simulink model "Lab_4"  (Simulink 9.1)
settings: Solver=VariableStepAuto  StartTime=0.0  StopTime=simulation_time  MaxStep=0.1
values from neighbouring files (symbols this model uses):
  a = (r_a + r_p)/2    (= 7178)    [main.m]
  i = 0    [main.m]
  I_1 = 0.0109    [main.m]
  I_2 = 0.0504    [main.m]
  I_3 = 0.055    [main.m]
  mu = 398600    [main.m]
  OMG = 0    [main.m]
  omg = 0    [main.m]
  phi_0 = 0    [main.m]
  psi_0 = 0    [main.m]
  q_c = [0; 1; 0; 0]    [main.m]
  theta = 0    [main.m]
  theta_0 = 0    [main.m]
  w1_0 = 0.02    [main.m]
  w2_0 = 0.01    [main.m]
  w3_0 = 0.05    [main.m]
undefined symbols (not defined in the file or in its folder): DCM_0, q_0
libraries: dspmathops x2, sharedutil x1
settings Model: SuppressorTable=22 serialization::archive 11 0 6 0 0 0 1 0  Creator=fcuzzocrea  LastModifiedBy=fcuzzocrea
settings DataIOCC: SaveFormat=Dataset
settings OptimizationCC: LifeSpan=auto
settings DebuggingCC: UnderspecifiedInitializationDetection=Simplified  MergeDetectMultiDrivingBlocksExec=error  SFUnexpectedBacktrackingDiag=error  SFNoUnconditionalDefaultTransitionDiag=error  SFExecutionAtInitializationDiag=warning
settings HardwareCC: ProdBitPerPointer=64  ProdBitPerSizeT=64  ProdBitPerPtrDiffT=64  ProdLargestAtomicFloat=Float  ProdIntDivRoundTo=Zero  ProdEndianess=LittleEndian  ProdWordSize=64  ProdHWDeviceType=Intel->x86-64 (Windows64)
settings ModelReferenceCC: PropagateSignalLabelsOutOfModel=on
settings CodeAppCC: StateflowObjectComments=off
settings GRTTargetCC: TargetLangStandard=C99 (ISO)  CombineOutputUpdateFcns=on  GRTInterface=off
settings ConfigComp: CovMetricSettings=dwe  CovHtmlReporting=off  CovSaveCumulativeToWorkspaceVar=off  CovSaveSingleToWorkspaceVar=off  CovExternalEMLEnable=on

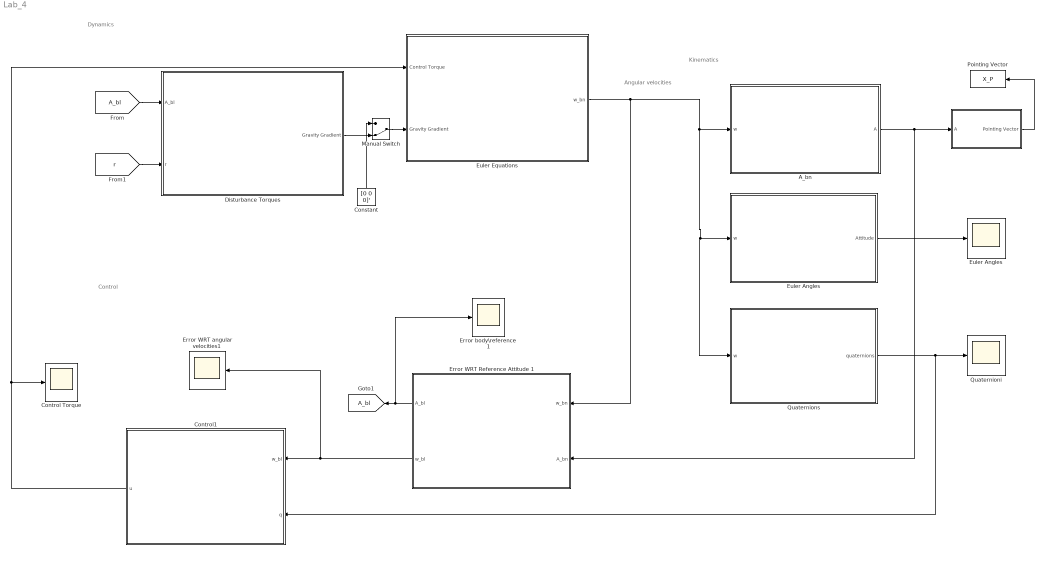
== system Lab_4 ==
  note: Dynamics
  note: Kinematics
  note: Angular velocities
  note: Control
  " " : Subsystem
  A_bn : Subsystem
  Constant : Constant  Value=[0 0 0]'
  "Control Torque " : Scope
  Control1 : Subsystem
  Disturbance Torques : Subsystem
  Error WRT Reference Attitude 1 : Subsystem
  Error WRT angular velocities1 : Scope
  Error body\reference  1 : Scope
  "Euler Angles " : Subsystem
  "Euler Angles  " : Scope
  "Euler Equations " : Subsystem
  Manual Switch : ManualSwitch  CurrentSetting=0
  "Pointing Vector " : ToWorkspace  VariableName=X_P  SampleTime=-1
  "Quaternioni " : Scope
  Quaternions : Subsystem
  tag scope: A_bl=global
  wires:
  " "/1("Pointing Vector ") -> "Pointing Vector "/1
  "Euler Angles "/1(Attitude) -> "Euler Angles  "/1
  [A_bl] -> Disturbance Torques/1(A_bl)
  [r] -> Disturbance Torques/2(r)
  Manual Switch/1 -> "Euler Equations "/2(Gravity Gradient)
  Constant/1 -> Manual Switch/1
  Disturbance Torques/1("Gravity Gradient ") -> Manual Switch/2
  Error WRT Reference Attitude 1/2(w_bl) -> Error WRT angular velocities1/1, Control1/1(w_bl)
  Quaternions/1(quaternions) -> Control1/2(q), "Quaternioni "/1
  A_bn/1(A) -> Error WRT Reference Attitude 1/2(A_bn), " "/1(A)
  Error WRT Reference Attitude 1/1(A_bl) -> Error body\reference  1/1, [A_bl]
  "Euler Equations "/1(w_bn) -> Error WRT Reference Attitude 1/1(w_bn), A_bn/1(w), Quaternions/1(w), "Euler Angles "/1(w)
  Control1/1(u) -> "Euler Equations "/1(Control Torque), "Control Torque "/1

== system Lab_4/  ==
  A : Inport
  Constant3 : Constant  Value=[1 0 0]'  VectorParams1D=off
  Math Function : Math  Operator=transpose  SaturateOnIntegerOverflow=on
  Product1 : Product  Multiplication=Matrix(*)
  "Pointing Vector " : Outport
  wires:
  Constant3/1 -> Product1/2
  Math Function/1 -> Product1/1
  A/1 -> Math Function/1
  Product1/1 -> "Pointing Vector "/1

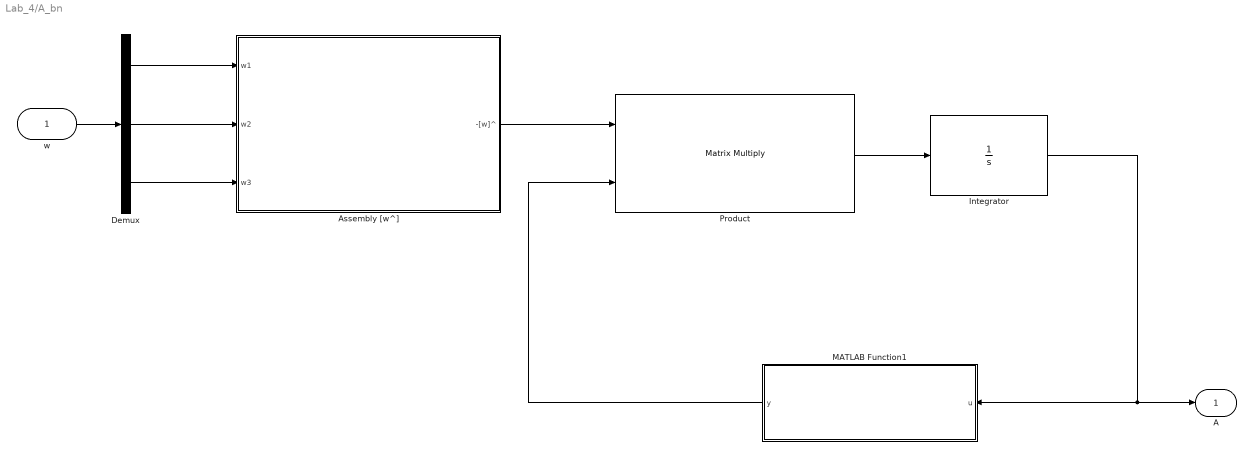
== system Lab_4/A_bn ==
  w : Inport  Unit=rad/s  PortDimensions=3
  "Assembly [w^] " : Subsystem
  Demux : Demux  Outputs=3
  Integrator : Integrator  InitialCondition=DCM_0
  MATLAB Function1 : MATLAB Function  TreatAsAtomicUnit=on
  Product : Product  Multiplication=Matrix(*)
  A : Outport
  wires:
  Product/1 -> Integrator/1
  Integrator/1 -> A/1, MATLAB Function1/1(u)
  w/1 -> Demux/1
  Demux/1 -> "Assembly [w^] "/1(w1)
  Demux/2 -> "Assembly [w^] "/2(w2)
  Demux/3 -> "Assembly [w^] "/3(w3)
  "Assembly [w^] "/1(-[w]^) -> Product/1
  MATLAB Function1/1(y) -> Product/2

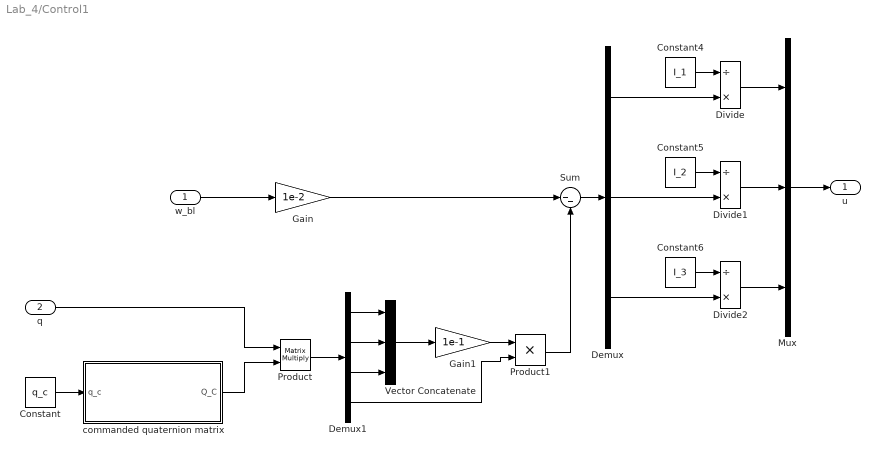
== system Lab_4/Control1 ==
  w_bl : Inport
  q : Inport  Port=2
  Constant : Constant  Value=q_c
  Constant4 : Constant  Value=I_1
  Constant5 : Constant  Value=I_2
  Constant6 : Constant  Value=I_3
  Demux : Demux  Outputs=3
  Demux1 : Demux
  Divide : Product  Inputs=/*
  Divide1 : Product  Inputs=/*
  Divide2 : Product  Inputs=/*
  Gain : Gain  Gain=1e-2
  Gain1 : Gain  Gain=1e-1
  Mux : Mux  Inputs=3
  Product : Product  Multiplication=Matrix(*)
  Product1 : Product
  Sum : Sum  Inputs=|--
  Vector Concatenate : Concatenate  NumInputs=3
  commanded quaternion matrix : MATLAB Function  TreatAsAtomicUnit=on
  u : Outport
  wires:
  w_bl/1 -> Gain/1
  Divide/1 -> Mux/1
  Constant4/1 -> Divide/1
  Constant5/1 -> Divide1/1
  Divide1/1 -> Mux/2
  Constant6/1 -> Divide2/1
  Divide2/1 -> Mux/3
  Demux/2 -> Divide1/2
  Demux/1 -> Divide/2
  Mux/1 -> u/1
  Demux/3 -> Divide2/2
  Constant/1 -> commanded quaternion matrix/1(q_c)
  q/1 -> Product/1
  commanded quaternion matrix/1(Q_C) -> Product/2
  Gain/1 -> Sum/1
  Sum/1 -> Demux/1
  Product/1 -> Demux1/1
  Demux1/4 -> Product1/2
  Demux1/1 -> Vector Concatenate/1
  Demux1/2 -> Vector Concatenate/2
  Demux1/3 -> Vector Concatenate/3
  Vector Concatenate/1 -> Gain1/1
  Gain1/1 -> Product1/1
  Product1/1 -> Sum/2

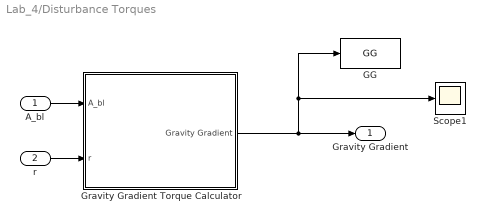
== system Lab_4/Disturbance Torques ==
  A_bl : Inport
  r : Inport  Port=2
  GG : ToWorkspace  VariableName=GG  SampleTime=-1
  Gravity Gradient Torque Calculator : Subsystem
  Scope1 : Scope
  "Gravity Gradient " : Outport
  wires:
  A_bl/1 -> Gravity Gradient Torque Calculator/1(A_bl)
  r/1 -> Gravity Gradient Torque Calculator/2(r)
  Gravity Gradient Torque Calculator/1(Gravity Gradient) -> Scope1/1, GG/1, "Gravity Gradient "/1

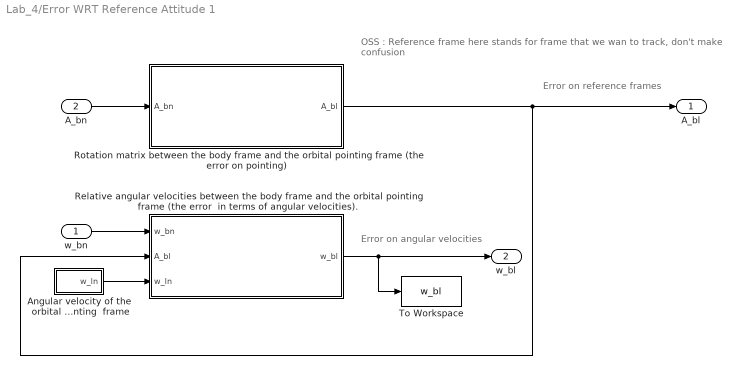
== system Lab_4/Error WRT Reference Attitude 1 ==
  note: Error on angular velocities
  note: Error on reference frames
  note: OSS : Reference frame here stands for frame that we wan to track, don't make confusion
  w_bn : Inport
  A_bn : Inport  Port=2
  Angular velocity of the  orbital pointing  frame : Subsystem
  Relative angular velocities between the body frame and the orbital pointing frame (the error  in terms of angular velocities). : Subsystem
  Rotation matrix between the body frame and the orbital pointing frame (the error on pointing) : Subsystem
  To Workspace : ToWorkspace  VariableName=w_bl  SampleTime=-1
  A_bl : Outport
  w_bl : Outport  Port=2
  wires:
  A_bn/1 -> Rotation matrix between the body frame and the orbital pointing frame (the error on pointing)/1("A_bn ")
  w_bn/1 -> Relative angular velocities between the body frame and the orbital pointing frame (the error  in terms of angular velocities)./1(w_bn)
  Rotation matrix between the body frame and the orbital pointing frame (the error on pointing)/1("A_bl   ") -> A_bl/1, Relative angular velocities between the body frame and the orbital pointing frame (the error  in terms of angular velocities)./2("A_bl ")
  Angular velocity of the  orbital pointing  frame/1(w_ln) -> Relative angular velocities between the body frame and the orbital pointing frame (the error  in terms of angular velocities)./3("w_ln ")
  Relative angular velocities between the body frame and the orbital pointing frame (the error  in terms of angular velocities)./1(w_bl) -> To Workspace/1, w_bl/1

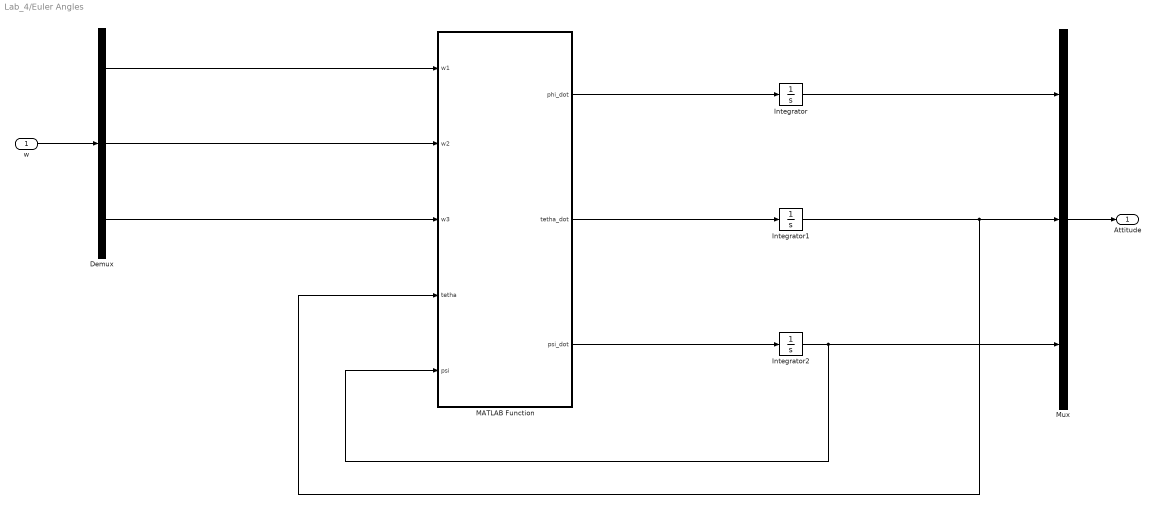
== system Lab_4/Euler Angles  ==
  w : Inport
  Demux : Demux  Outputs=3
  Integrator : Integrator  InitialCondition=phi_0
  Integrator1 : Integrator  InitialCondition=theta_0
  Integrator2 : Integrator  InitialCondition=psi_0
  MATLAB Function : MATLAB Function  TreatAsAtomicUnit=on
  Mux : Mux  Inputs=3
  Attitude : Outport
  wires:
  Demux/1 -> MATLAB Function/1(w1)
  Demux/2 -> MATLAB Function/2(w2)
  Demux/3 -> MATLAB Function/3(w3)
  MATLAB Function/1(phi_dot) -> Integrator/1
  MATLAB Function/2(tetha_dot) -> Integrator1/1
  MATLAB Function/3(psi_dot) -> Integrator2/1
  Integrator/1 -> Mux/1
  Integrator1/1 -> Mux/2, MATLAB Function/4(tetha)
  Mux/1 -> Attitude/1
  Integrator2/1 -> MATLAB Function/5(psi), Mux/3
  w/1 -> Demux/1

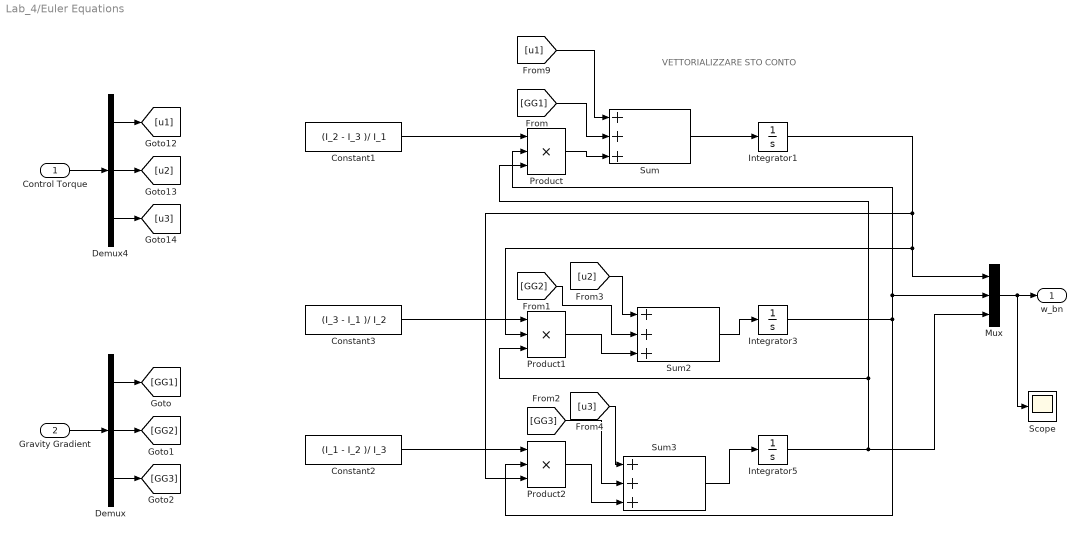
== system Lab_4/Euler Equations  ==
  note: VETTORIALIZZARE STO CONTO
  Control Torque : Inport
  Gravity Gradient : Inport  Port=2
  Constant1 : Constant  Value=(I_2 - I_3 )/ I_1
  Constant2 : Constant  Value=(I_1 - I_2 )/ I_3
  Constant3 : Constant  Value=(I_3 - I_1 )/ I_2
  Demux : Demux  Outputs=3
  Demux4 : Demux  Outputs=3
  Integrator1 : Integrator  InitialCondition=w1_0
  Integrator3 : Integrator  InitialCondition=w2_0
  Integrator5 : Integrator  InitialCondition=w3_0
  Mux : Mux  Inputs=3
  Product : Product  Inputs=3
  Product1 : Product  Inputs=3
  Product2 : Product  Inputs=3
  Scope : Scope
  Sum : Sum  Inputs=+++
  Sum2 : Sum  Inputs=+++
  Sum3 : Sum  Inputs=+++
  w_bn : Outport
  wires:
  Integrator3/1 -> Product2/2, Mux/2, Product/2
  Integrator5/1 -> Mux/3, Product/3, Product1/3
  Constant1/1 -> Product/1
  Constant3/1 -> Product1/1
  Constant2/1 -> Product2/1
  Integrator1/1 -> Product1/2, Mux/1, Product2/3
  Mux/1 -> Scope/1, w_bn/1
  Sum/1 -> Integrator1/1
  Sum2/1 -> Integrator3/1
  Sum3/1 -> Integrator5/1
  Gravity Gradient/1 -> Demux/1
  Demux/1 -> [GG1]
  Demux/2 -> [GG2]
  Demux/3 -> [GG3]
  Demux4/2 -> [u2]
  Control Torque/1 -> Demux4/1
  Demux4/3 -> [u3]
  Demux4/1 -> [u1]
  Product/1 -> Sum/3
  [GG1] -> Sum/2
  [u1] -> Sum/1
  Product1/1 -> Sum2/3
  [GG2] -> Sum2/2
  [u2] -> Sum2/1
  Product2/1 -> Sum3/3
  [GG3] -> Sum3/2
  [u3] -> Sum3/1

== system Lab_4/Quaternions ==
  w : Inport
  Integrator2 : Integrator  InitialCondition=q_0
  Quaternion kinematics : MATLAB Function  TreatAsAtomicUnit=on
  quaternions : Outport
  wires:
  Integrator2/1 -> quaternions/1, Quaternion kinematics/1(q)  "q"
  Quaternion kinematics/1(dq) -> Integrator2/1  "dq"
  w/1 -> Quaternion kinematics/2(omega)  "ω_b"

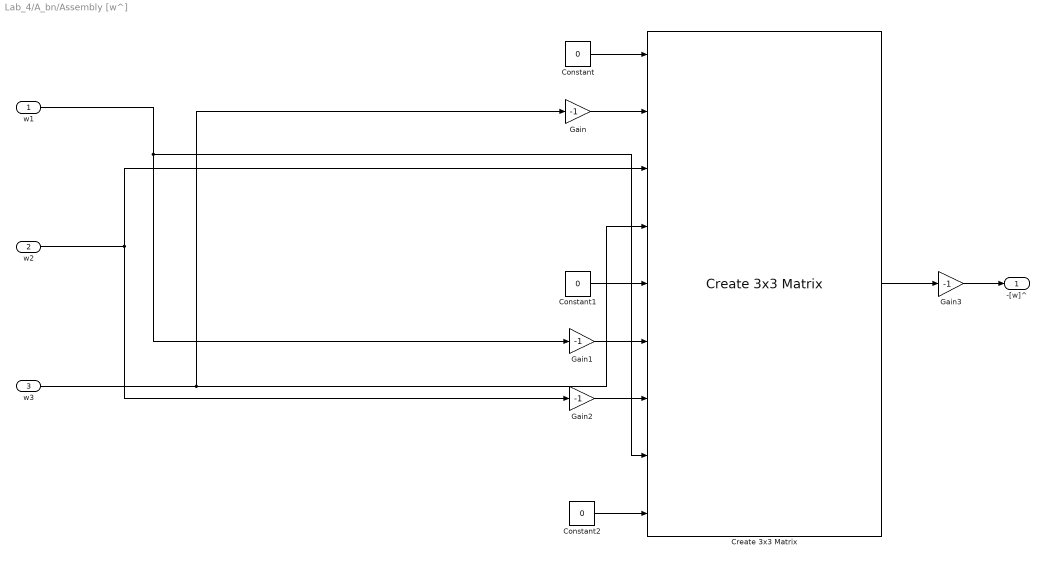
== system Lab_4/A_bn/Assembly [w^]  ==
  w1 : Inport
  w2 : Inport  Port=2
  w3 : Inport  Port=3
  Constant : Constant  Value=0
  Constant1 : Constant  Value=0
  Constant2 : Constant  Value=0
  Create 3x3 Matrix : sharedutil/Create 3x3 Matrix
  Gain{,1..3} (4 alike) : Gain  Gain=-1
  -[w]^ : Outport
  wires:
  Gain2/1 -> Create 3x3 Matrix/7
  Gain1/1 -> Create 3x3 Matrix/6
  w1/1 -> Create 3x3 Matrix/8, Gain1/1
  w3/1 -> Create 3x3 Matrix/4, Gain/1
  Constant1/1 -> Create 3x3 Matrix/5
  Constant2/1 -> Create 3x3 Matrix/9
  Constant/1 -> Create 3x3 Matrix/1
  w2/1 -> Gain2/1, Create 3x3 Matrix/3
  Gain/1 -> Create 3x3 Matrix/2
  Create 3x3 Matrix/1 -> Gain3/1
  Gain3/1 -> -[w]^/1

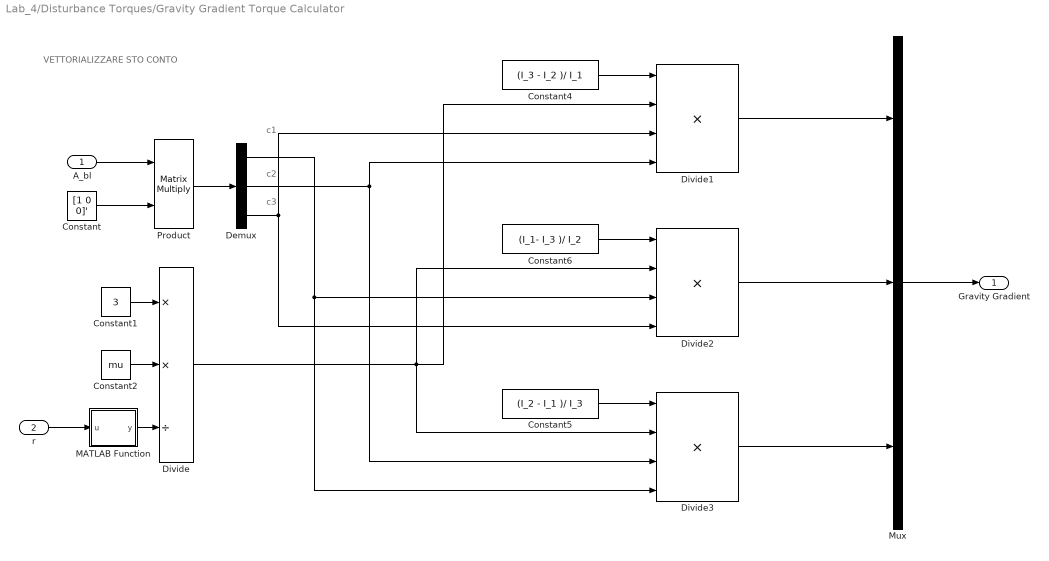
== system Lab_4/Disturbance Torques/Gravity Gradient Torque Calculator ==
  note: VETTORIALIZZARE STO CONTO
  note: c2
  note: c3
  note: c1
  A_bl : Inport
  r : Inport  Port=2
  Constant : Constant  Value=[1 0 0]'
  Constant1 : Constant  Value=3
  Constant2 : Constant  Value=mu
  Constant4 : Constant  Value=(I_3 - I_2 )/ I_1
  Constant5 : Constant  Value=(I_2 - I_1 )/ I_3
  Constant6 : Constant  Value=(I_1- I_3 )/ I_2
  Demux : Demux  Outputs=3
  Divide : Product  Inputs=**/
  Divide1 : Product  Inputs=****
  Divide2 : Product  Inputs=****
  Divide3 : Product  Inputs=****
  MATLAB Function : MATLAB Function  TreatAsAtomicUnit=on
  Mux : Mux  Inputs=3
  Product : Product  Multiplication=Matrix(*)
  Gravity Gradient : Outport
  wires:
  Demux/3 -> Divide2/4, Divide1/3
  Constant1/1 -> Divide/1
  r/1 -> MATLAB Function/1(u)
  Constant5/1 -> Divide3/1
  Divide/1 -> Divide3/2, Divide1/2, Divide2/2
  Demux/1 -> Divide3/4, Divide2/3
  Demux/2 -> Divide3/3, Divide1/4
  Product/1 -> Demux/1
  Constant6/1 -> Divide2/1
  A_bl/1 -> Product/1
  Constant4/1 -> Divide1/1
  MATLAB Function/1(y) -> Divide/3
  Constant/1 -> Product/2
  Constant2/1 -> Divide/2
  Divide1/1 -> Mux/1
  Divide2/1 -> Mux/2
  Divide3/1 -> Mux/3
  Mux/1 -> Gravity Gradient/1

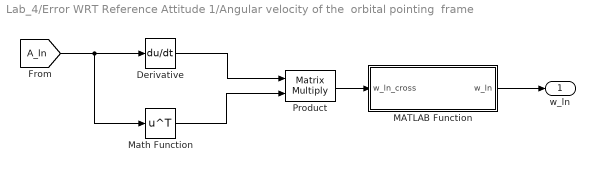
== system Lab_4/Error WRT Reference Attitude 1/Angular velocity of the  orbital pointing  frame ==
  Derivative : Derivative
  MATLAB Function : MATLAB Function  TreatAsAtomicUnit=on
  Math Function : Math  Operator=transpose  SaturateOnIntegerOverflow=on
  Product : Product  Multiplication=Matrix(*)
  w_ln : Outport
  wires:
  [A_ln] -> Math Function/1, Derivative/1
  Math Function/1 -> Product/2
  Derivative/1 -> Product/1
  Product/1 -> MATLAB Function/1(w_ln_cross)
  MATLAB Function/1(w_ln) -> w_ln/1

== system Lab_4/Error WRT Reference Attitude 1/Relative angular velocities between the body frame and the orbital pointing frame (the error  in terms of angular velocities). ==
  w_bn : Inport
  "A_bl " : Inport  Port=2
  "w_ln " : Inport  Port=3
  Product : Product  Multiplication=Matrix(*)
  Subtract : Sum  Inputs=+-
  w_bl : Outport
  wires:
  Product/1 -> Subtract/2
  Subtract/1 -> w_bl/1
  w_bn/1 -> Subtract/1
  "A_bl "/1 -> Product/1
  "w_ln "/1 -> Product/2

== system Lab_4/Error WRT Reference Attitude 1/Rotation matrix between the body frame and the orbital pointing frame (the error on pointing) ==
  note: NB : La DCM è A_bn, per cui moltiplicando A_ln * A_bn becco A_bl !!!!
  note: Reference Attitude
  "A_bn " : Inport
  Math Function1 : Math  Operator=transpose  SaturateOnIntegerOverflow=on
  Product : Product  Multiplication=Matrix(*)
  Rotation matrix between the  pointing orbital frame and the inertial frame : Subsystem
  "A_bl   " : Outport
  wires:
  "A_bn "/1 -> Product/1
  Rotation matrix between the  pointing orbital frame and the inertial frame/1("A_L\\N ") -> Math Function1/1
  Product/1 -> "A_bl   "/1
  Math Function1/1 -> Product/2

== system Lab_4/Error WRT Reference Attitude 1/Rotation matrix between the body frame and the orbital pointing frame (the error on pointing)/Rotation matrix between the  pointing orbital frame and the inertial frame ==
  Full Orbital Dynamics : Subsystem
  Initial Conditions (KEP) : Constant  Value=[a, e, i, OMG, omg, theta]
  Planetary Constant : Constant  Value=mu
  "A_L\\N " : Outport
  tag scope: A_ln=global
  wires:
  Planetary Constant/1 -> Full Orbital Dynamics/1(mu)
  Initial Conditions (KEP)/1 -> Full Orbital Dynamics/2(Initial Condition (kep))
  Full Orbital Dynamics/1(A_L\N) -> [A_ln], "A_L\\N "/1

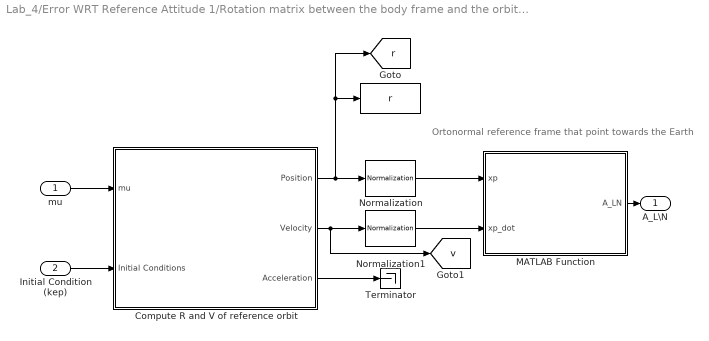
== system Lab_4/Error WRT Reference Attitude 1/Rotation matrix between the body frame and the orbital pointing frame (the error on pointing)/Rotation matrix between the  pointing orbital frame and the inertial frame/Full Orbital Dynamics ==
  note: Ortonormal reference frame that point towards the Earth
  mu : Inport
  Initial Condition (kep) : Inport  Port=2
  "  " : ToWorkspace  VariableName=r  SampleTime=-1
  Compute R and V of reference orbit : Subsystem
  MATLAB Function : MATLAB Function  TreatAsAtomicUnit=on
  Normalization : dspmathops/Normalization  NormType=2-norm  Bias=1e-10  NormOver=Each row  Dimension=1  outputDataTypeStr=Inherit: Same as product output  outputLastDataTypeStr=Inherit: Same as product output  outputMin=[]  outputMax=[]  accumDataTypeStr=Inherit: Same as product output  accumLastDataTypeStr=Inherit: Same as product output  roundingMode=Floor  overflowMode=off
      settings: SourceProductName=DSP System Toolbox
  Normalization1 : dspmathops/Normalization  NormType=2-norm  Bias=1e-10  NormOver=Each row  Dimension=1  outputDataTypeStr=Inherit: Same as product output  outputLastDataTypeStr=Inherit: Same as product output  outputMin=[]  outputMax=[]  accumDataTypeStr=Inherit: Same as product output  accumLastDataTypeStr=Inherit: Same as product output  roundingMode=Floor  overflowMode=off
      settings: SourceProductName=DSP System Toolbox
  Terminator : Terminator
  A_L\N : Outport
  tag scope: r=global, v=global
  wires:
  mu/1 -> Compute R and V of reference orbit/1(mu)
  Initial Condition (kep)/1 -> Compute R and V of reference orbit/2(Initial Conditions)
  Compute R and V of reference orbit/1(Position) -> [r], "  "/1, Normalization/1
  Compute R and V of reference orbit/2(Velocity) -> [v], Normalization1/1
  Compute R and V of reference orbit/3(Acceleration) -> Terminator/1
  Normalization/1 -> MATLAB Function/1(xp)
  MATLAB Function/1(A_LN) -> A_L\N/1
  Normalization1/1 -> MATLAB Function/2(xp_dot)

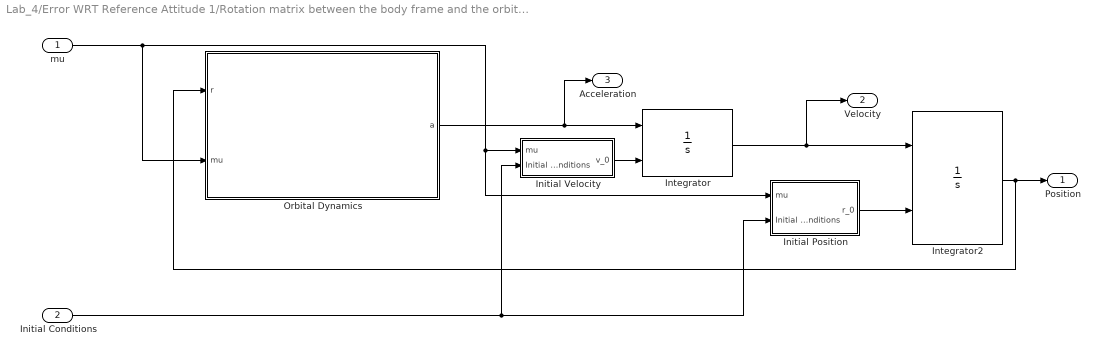
== system Lab_4/Error WRT Reference Attitude 1/Rotation matrix between the body frame and the orbital pointing frame (the error on pointing)/Rotation matrix between the  pointing orbital frame and the inertial frame/Full Orbital Dynamics/Compute R and V of reference orbit ==
  mu : Inport
  Initial Conditions : Inport  Port=2
  Initial Position : Subsystem
  Initial Velocity : Subsystem
  Integrator : Integrator  InitialConditionSource=external  InitialCondition=[r,v]=kep2car(kep,mu);  ContinuousStateAttributes='velocity'
  Integrator2 : Integrator  InitialConditionSource=external  InitialCondition=[r,v]=kep2car(kep,mu);  ContinuousStateAttributes='position'
  Orbital Dynamics : MATLAB Function  TreatAsAtomicUnit=on
  Position : Outport
  Velocity : Outport  Port=2
  Acceleration : Outport  Port=3
  wires:
  Initial Conditions/1 -> Initial Position/2(Initial Conditions), Initial Velocity/2(Initial Conditions)
  Initial Position/1(r_0) -> Integrator2/2
  Initial Velocity/1(v_0) -> Integrator/2
  Orbital Dynamics/1(a) -> Acceleration/1, Integrator/1
  Integrator/1 -> Velocity/1, Integrator2/1
  mu/1 -> Initial Position/1(mu), Initial Velocity/1(mu), Orbital Dynamics/2(mu)
  Integrator2/1 -> Orbital Dynamics/1(r), Position/1

== system Lab_4/Error WRT Reference Attitude 1/Rotation matrix between the body frame and the orbital pointing frame (the error on pointing)/Rotation matrix between the  pointing orbital frame and the inertial frame/Full Orbital Dynamics/Compute R and V of reference orbit/Initial Position ==
  mu : Inport
  Initial Conditions : Inport  Port=2
  MATLAB Function2 : MATLAB Function  TreatAsAtomicUnit=on
  r_0 : Outport
  wires:
  MATLAB Function2/1(r_0) -> r_0/1
  mu/1 -> MATLAB Function2/2(mu)
  Initial Conditions/1 -> MATLAB Function2/1(kep)

== system Lab_4/Error WRT Reference Attitude 1/Rotation matrix between the body frame and the orbital pointing frame (the error on pointing)/Rotation matrix between the  pointing orbital frame and the inertial frame/Full Orbital Dynamics/Compute R and V of reference orbit/Initial Velocity ==
  mu : Inport
  Initial Conditions : Inport  Port=2
  MATLAB Function1 : MATLAB Function  TreatAsAtomicUnit=on
  v_0 : Outport
  wires:
  MATLAB Function1/1(v_0) -> v_0/1
  mu/1 -> MATLAB Function1/2(mu)
  Initial Conditions/1 -> MATLAB Function1/1(kep)

== matlab function Euler Angles /MATLAB Function ==
  data: phi_dot output double; tetha_dot output double; psi_dot output double; w1 input double; w2 input double; w3 input double; tetha input double; psi input double
function [phi_dot,tetha_dot, psi_dot] = euler_eqtns(w1,w2,w3, tetha, psi)

% Euler rotations (sequence 123)
phi_dot = 1/cos(tetha)*((w1*cos(psi)-w2*sin(psi)));
tetha_dot = (w2*cos(psi))+(w1*sin(psi));
psi_dot = w3 - ((w1*cos(psi) - w2*sin(psi))*(sin(tetha)/cos(tetha)));

end

== matlab function Quaternions/Quaternion kinematics ==
  data: q input double size=4; dq output double size=4; omega input double size=3
function dq = quat_kin(q, omega)
%#codegen
qnorm = sqrt(q(1)^2 + q(2)^2 + q(3)^2 + q(4)^2);
q = q./qnorm;
W = [ q(4) -q(3)  q(2) ;
      q(3)  q(4) -q(1) ;
     -q(2)  q(1)  q(4) ; 
     -q(1) -q(2) -q(3)];

dq = 0.5 * W * omega;

== matlab function A_bn/MATLAB Function1 ==
  data: u input double; y output double
function y = ortonormalize(u)

y = u.*3/2 - u*u'*(u./2);

y = u;

end

== matlab function Disturbance Torques/Gravity Gradient Torque Calculator/MATLAB Function ==
  data: u input double; y output double
function y = norm3(u)

y = (norm(u))^3;

end

== matlab function Control1/commanded quaternion matrix ==
  data: Q_C output double; q_c input double
function Q_C  = command_quaternion (q_c)
%#codegen

Q_C = [ q_c(4)  q_c(3)  -q_c(2) -q_c(1) ;
       -q_c(3)  q_c(4)   q_c(1) -q_c(2) ;
        q_c(2) -q_c(1)   q_c(4) -q_c(3) ; 
        q_c(1)  q_c(2)   q_c(3)  q_c(4) ];

end

== matlab function Error WRT Reference Attitude 1/Angular velocity of the orbital pointing frame/MATLAB Function ==
  data: w_ln_cross input double; w_ln output double
function w_ln = w_component_extractor(w_ln_cross)

w_1 = w_ln_cross(3,2);
w_2 = w_ln_cross(1,3);
w_3 = w_ln_cross(2,1);

w_ln = [w_1, w_2, w_3]';
end

== matlab function Error WRT Reference Attitude 1/Rotation matrix between the body frame and the orbital pointing frame (the error on pointing)/Rotation matrix between the pointing orbital frame and the inertial frame/Full Orbital Dynamics/Compute R and V of reference orbit/Initial Position/MATLAB Function2 ==
  data: r_0 output double; kep input double; mu input double
function r_0  = kep2car(kep,mu)

% Using kep2car function to find position and velocity at initial condition
[r_0,~]=kep2car(kep,mu);

end

== matlab function Error WRT Reference Attitude 1/Rotation matrix between the body frame and the orbital pointing frame (the error on pointing)/Rotation matrix between the pointing orbital frame and the inertial frame/Full Orbital Dynamics/Compute R and V of reference orbit/Initial Velocity/MATLAB Function1 ==
  data: v_0 output double; kep input double; mu input double
function v_0  = kep2car(kep,mu)

% Using kep2car function to find velocity at initial condition
[~,v_0]=kep2car(kep,mu);

end

== matlab function Error WRT Reference Attitude 1/Rotation matrix between the body frame and the orbital pointing frame (the error on pointing)/Rotation matrix between the pointing orbital frame and the inertial frame/Full Orbital Dynamics/Compute R and V of reference orbit/Orbital Dynamics ==
  data: r input double; a output double; mu input double
function a  = orbit_equation(r,mu)

rn = norm(r);

a = -(mu/norm(r)^3)*r;

end

== matlab function Error WRT Reference Attitude 1/Rotation matrix between the body frame and the orbital pointing frame (the error on pointing)/Rotation matrix between the pointing orbital frame and the inertial frame/Full Orbital Dynamics/MATLAB Function ==
  data: xp input double; A_LN output double; xp_dot input double
function A_LN = assembly_ALN(xp,xp_dot)

xp = xp';
xp_dot = xp_dot';

r_1 = xp;                                           % Points toward the Earth
r_2 = (cross(xp_dot,xp))/(norm(cross(xp_dot,xp)));  % Points toward angular momentum vector
r_3 = cross(r_1,r_2);                               % To be ortoghonal

A_LN = [r_1; r_3; r_2];                             % BE CONSISTENT WITH THE ACTUAL REFERENCE SYSTEM USED TO COMPUTE R AND V
                                                    % ACTUALLY FOR ME :
                                                    %    
                                                    %      x = direction of the vector pointing to earth    
                                                    %
                                                    %      z = direction of the out of plane vector     
                                                    %      
                                                    %      y = third vector
                                                    %

end
